simulink model "stepper_tfn"  (R2016a)
settings: Solver=ode4  StartTime=0.0  StopTime=245  RelTol=1e-3
undefined symbols (not defined in the file): c, D, J
libraries: dspswit3 x3
settings Model: Creator=shohei  LastModifiedBy=shohei

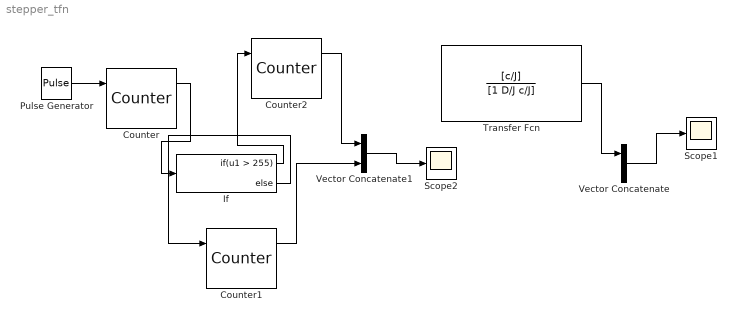
== system stepper_tfn ==
  Counter : dspswit3/Counter  Direction=Up  CountEvent=Rising edge  CounterSize=User defined  MaxCount=1023  InitialCount=0  Output=Count and Hit  HitValue=32  ResetInput=on  SamplesPerFrame=1  Ts=1  CntDtype=double  HitDtype=Logical
  Counter1 : dspswit3/Counter  Direction=Down  CountEvent=Rising edge  CounterSize=User defined  MaxCount=1023  InitialCount=0  Output=Count and Hit  HitValue=32  ResetInput=on  SamplesPerFrame=1  Ts=1  CntDtype=double  HitDtype=Logical
  Counter2 : dspswit3/Counter  Direction=Up  CountEvent=Rising edge  CounterSize=User defined  MaxCount=1023  InitialCount=0  Output=Count and Hit  HitValue=32  ResetInput=on  SamplesPerFrame=1  Ts=1  CntDtype=double  HitDtype=Logical
  If : If  IfExpression=u1 > 255
  Pulse Generator : DiscretePulseGenerator  PulseType=Time based  Period=0.08  PulseWidth=5
  Scope1 : Scope
  Scope2 : Scope
  Transfer Fcn : TransferFcn  Numerator=[c/J]  Denominator=[1 D/J c/J]
  Vector Concatenate : Concatenate
  Vector Concatenate1 : Concatenate
  wires:
  Vector Concatenate/1 -> Scope1/1
  Transfer Fcn/1 -> Vector Concatenate/1
  Pulse Generator/1 -> Counter/1
  Counter/1 -> If/1
  If/1 -> Counter2/1
  Counter1/1 -> Vector Concatenate1/2
  If/2 -> Counter1/1
  Counter2/1 -> Vector Concatenate1/1
  Vector Concatenate1/1 -> Scope2/1
